simulink library "ClusterLibrary"  (R2023b)
settings: Solver=VariableStepAuto  StartTime=0.0  StopTime=10.0  RelTol=1e-3
undefined symbols (not defined in the file or in its folder): DiscIntNeverNeededParam
libraries: simulink x1
settings Model: Creator=joel  LastModifiedBy=joel

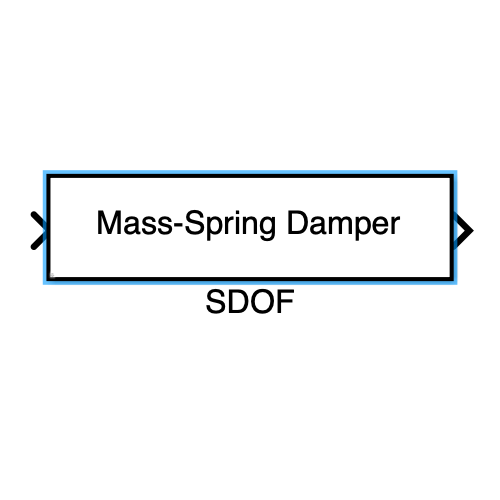
[thumbnail: Simulink's stored preview of the top-level diagram]
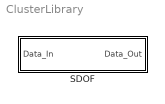
== system ClusterLibrary ==
  SDOF : Subsystem  TreatAsAtomicUnit=on  mask{MassConstant=.3, SpringConstant=20, DampingConstant=3}
      mask prompts: MassConstant "Mass Value"; SpringConstant "Spring Rate"; DampingConstant "Damper Rate"
      mask DialogControl DescTextVar Prompt: This is a single degree of freedom mass spring damper, allowing for a spring effect on the output, based on the input value
      mask Display: disp('Mass-Spring Damper');

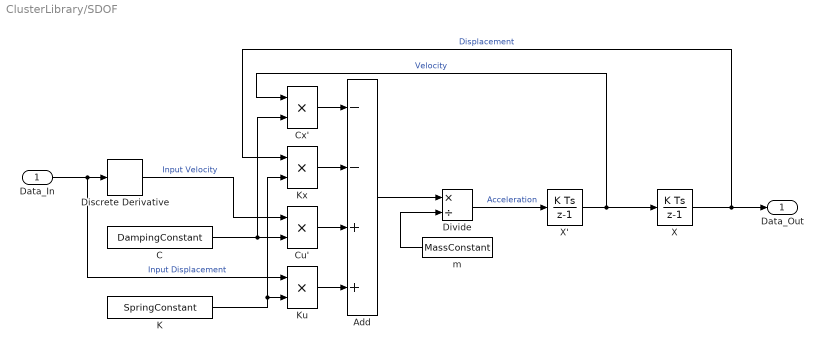
== system ClusterLibrary/SDOF ==
  Data_In : Inport
  Add : Sum  Inputs=--++
  C : Constant  Value=DampingConstant
  Cu' : Product
  Cx' : Product
  Discrete Derivative : simulink/Discrete/Discrete Derivative  gainval=1.0  ICPrevScaledInput=0.0  OutMin=[]  OutMax=[]  OutDataType=fixdt(1, 16)  OutScaling=2^-10  DoSatur=off
  Divide : Product  Inputs=*/
  K : Constant  Value=SpringConstant
  Ku : Product
  Kx : Product
  X : DiscreteIntegrator  SampleTime=-1  OutDataTypeStr=Inherit: Inherit via back propagation  ICPrevOutput=DiscIntNeverNeededParam  ICPrevScaledInput=DiscIntNeverNeededParam
  X' : DiscreteIntegrator  SampleTime=-1  ICPrevOutput=DiscIntNeverNeededParam  ICPrevScaledInput=DiscIntNeverNeededParam
  m : Constant  Value=MassConstant
  Data_Out : Outport
  wires:
  Cx'/1 -> Add/1
  Kx/1 -> Add/2
  C/1 -> Cx'/2, Cu'/2
  X/1 -> Data_Out/1, Kx/1  "Displacement"
  Add/1 -> Divide/1
  m/1 -> Divide/2
  Ku/1 -> Add/4
  Cu'/1 -> Add/3
  K/1 -> Kx/2, Ku/2
  Divide/1 -> X'/1  "Acceleration"
  X'/1 -> Cx'/1, X/1  "Velocity"
  Discrete Derivative/1 -> Cu'/1  "Input Velocity"
  Data_In/1 -> Discrete Derivative/1, Ku/1  "Input Displacement"
